simulink model "gm_combinedTxRx_ExternalMode"  (R2017b)
settings: Solver=FixedStepDiscrete  StartTime=0.0  StopTime=10.0  RelTol=1e-3
InitFcn:
  | modelSettings
undefined symbols (not defined in the file or in its folder): coeff, filt, j, RadioSampleRate, VibertiTracebackLength, xPreambleSeq
libraries: simulink x20, dsphdlfiltering x20, hdlsllib x10, hdlmdlgenlib x6, dspsigops x5, commseqgen3 x4, commdigbbndpm3 x3, commcrc2 x2, commcnvcod2 x2, commsource2 x1, dspstat3 x1, dspmlti4 x1
(part 2 of 5)

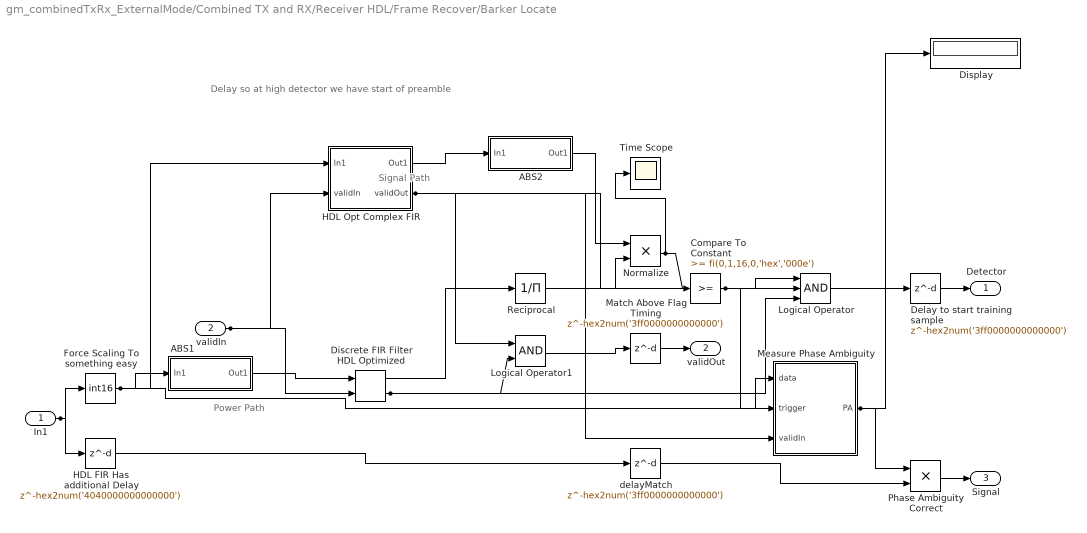
== system gm_combinedTxRx_ExternalMode/Combined TX and RX/Receiver HDL/Frame Recover/Barker Locate ==
  note: Signal Path
  note: Power Path
  note: Delay so at high detector we have start of preamble
  In1 : Inport  PortDimensions=1  SampleTime=1e-06
  validIn : Inport  Port=2  PortDimensions=1  SampleTime=1e-06
  ABS1 : Subsystem
  ABS2 : Subsystem
  Compare To Constant : simulink/Logic and Bit Operations/Compare To Constant  relop=>=  const=fi(0,1,16,0,'hex','000e')  OutDataTypeStr=boolean
  "Delay to start training sample " : Delay  DelayLength=hex2num('3ff0000000000000')  InitialCondition=0  InputProcessing=Inherited  SampleTime=1e-06
  Discrete FIR Filter HDL Optimized : dsphdlfiltering/Discrete FIR Filter HDL Optimized  Numerator=ones(1,length(xPreambleSeq)*1)/1  Sharing=off  SharingFactor=2  SimulateUsing=Code generation  roundingMode=Floor  overflowMode=off  CoefficientsDataTypeStr=Inherit: Same word length as input  CoefficientsMin=[]  CoefficientsMax=[]  OutputDataTypeStr=fixdt(1,17,0)  OutputMin=[]  OutputMax=[]  ValidInPort=on  ReadyPort=off
      settings: SourceProductName=DSP System Toolbox  SourceProductBaseCode=DS
  Display : Display
  Force Scaling To something easy : DataTypeConversion  OutDataTypeStr=int16  SampleTime=1e-06  SaturateOnIntegerOverflow=on
  HDL FIR Has additional Delay : Delay  DelayLength=hex2num('4040000000000000')  InitialCondition=0  InputProcessing=Inherited  SampleTime=1e-06
  HDL Opt Complex FIR : Subsystem  mask{Taps=reshape([complex(-0.7071067811865477, -0.7071067811865475) complex(-0.7071067811865477, -0.7071067811865475) complex(-0.7071067811865477, -0.7071067811865475) complex(0.7071067811865476, 0.7071067811865476) complex(0.7071067811865476, 0.7071067811865476) complex(0.7071067811865476, 0.7071067811865476) complex(-0.7071067811865477, -0.7071067811865475) complex(0.7071067811865476, 0.7071067811865476) complex(-0.7071067811865477, -0.7071067811865475) complex(-0.7071067811865477, -0.7071067811865475) complex(0.7071067811865476, 0.7071067811865476) complex(-0.7071067811865477, -0.7071067811865475) complex(-0.7071067811865477, -0.7071067811865475) complex(-0.7071067811865477, -0.7071067811865475) complex(0.7071067811865476, 0.7071067811865476) complex(0.7071067811865476, 0.7071067811865476) complex(0.7071067811865476, 0.7071067811865476) complex(-0.7071067811865477, -0.7071067811865475) complex(0.7071067811865476, 0.7071067811865476) complex(-0.7071067811865477, -0.7071067811865475) complex(-0.7071067811865477, -0.7071067811865475) complex(0.7071067811865476, 0.7071067811865476) complex(-0.7071067811865477, -0.7071067811865475) complex(-0.7071067811865477, -0.7071067811865475) complex(-0.7071067811865477, -0.7071067811865475) complex(0.7071067811865476, 0.7071067811865476) complex(0.7071067811865476, 0.7071067811865476) complex(0.7071067811865476, 0.7071067811865476)].', [1  28])}
  Logical Operator : Logic  Inputs=3  AllPortsSameDT=off  OutDataTypeStr=boolean  SampleTime=1e-06
  Logical Operator1 : Logic  AllPortsSameDT=off  OutDataTypeStr=boolean  SampleTime=1e-06
  Match Above Flag Timing : Delay  DelayLength=hex2num('3ff0000000000000')  InitialCondition=0  InputProcessing=Inherited  SampleTime=1e-06
  Measure Phase Ambiguity : Subsystem
  Normalize : Product  Inputs=**  OutDataTypeStr=int16  RndMeth=Simplest  SampleTime=1e-06  SaturateOnIntegerOverflow=on
  Phase Ambiguity Correct : Product  Inputs=**  OutDataTypeStr=fixdt(1, 16, 14)  SampleTime=1e-06
  Reciprocal : Product  Inputs=/  OutDataTypeStr=fixdt(1, 17, 15)  SampleTime=1e-06  SaturateOnIntegerOverflow=on  RndMeth=Zero
  Time Scope : Scope
  delayMatch : Delay  DelayLength=hex2num('3ff0000000000000')  InitialCondition=0  InputProcessing=Inherited  SampleTime=1e-06
  Detector : Outport
  validOut : Outport  Port=2
  Signal : Outport  Port=3
  wires:
  ABS1/1(Out1) -> Discrete FIR Filter HDL Optimized/1
  ABS2/1(Out1) -> Normalize/1
  Compare To Constant/1 -> Logical Operator/1, Measure Phase Ambiguity/2(trigger)
  "Delay to start training sample "/1 -> Detector/1
  Discrete FIR Filter HDL Optimized/1 -> Reciprocal/1
  Discrete FIR Filter HDL Optimized/2 -> Logical Operator1/2, Logical Operator/3
  Force Scaling To something easy/1 -> ABS1/1(In1), HDL Opt Complex FIR/1(In1), Measure Phase Ambiguity/1(data)
  delayMatch/1 -> Phase Ambiguity Correct/2
  HDL Opt Complex FIR/1(Out1) -> ABS2/1(In1)
  HDL Opt Complex FIR/2(validOut) -> Logical Operator1/1, Logical Operator/2, Measure Phase Ambiguity/3(validIn)
  Logical Operator/1 -> "Delay to start training sample "/1
  Logical Operator1/1 -> Match Above Flag Timing/1
  Match Above Flag Timing/1 -> validOut/1
  Measure Phase Ambiguity/1(PA) -> Phase Ambiguity Correct/1, Display/1
  Normalize/1 -> Compare To Constant/1, Time Scope/1
  Phase Ambiguity Correct/1 -> Signal/1
  Reciprocal/1 -> Normalize/2
  In1/1 -> Force Scaling To something easy/1, HDL FIR Has additional Delay/1
  validIn/1 -> HDL Opt Complex FIR/2(validIn), Discrete FIR Filter HDL Optimized/2
  HDL FIR Has additional Delay/1 -> delayMatch/1

== system gm_combinedTxRx_ExternalMode/Combined TX and RX/Receiver HDL/Frame Recover/Enable Equalizer and Packet Decode (Latch) ==
  start : Inport  SampleTime=1e-06
  validIn : Inport  Port=2  SampleTime=1e-06
  RxTxFixedPointLibrary_c12_Enable_Equalizer_and_Packet_Decode__L : MATLAB Function  TreatAsAtomicUnit=on
  enable : Outport
  wires:
  RxTxFixedPointLibrary_c12_Enable_Equalizer_and_Packet_Decode__L/1(enable) -> enable/1
  start/1 -> RxTxFixedPointLibrary_c12_Enable_Equalizer_and_Packet_Decode__L/1(start)
  validIn/1 -> RxTxFixedPointLibrary_c12_Enable_Equalizer_and_Packet_Decode__L/2(validIn)

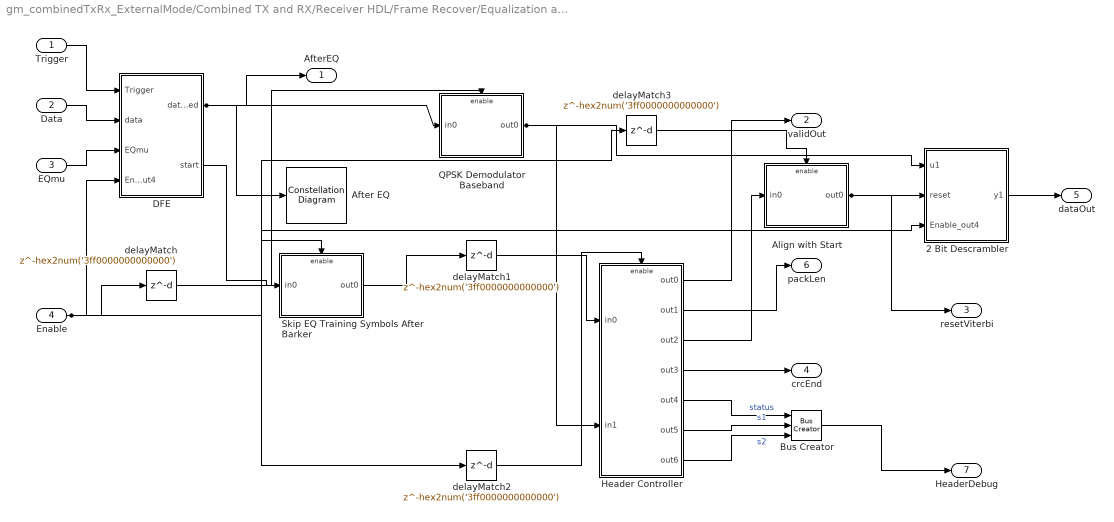
== system gm_combinedTxRx_ExternalMode/Combined TX and RX/Receiver HDL/Frame Recover/Equalization and Demodulation ==
  Trigger : Inport  SampleTime=1e-06
  Data : Inport  Port=2  SampleTime=1e-06
  EQmu : Inport  Port=3  SampleTime=1e-06
  Enable : Inport  Port=4  OutDataTypeStr=boolean  SampleTime=1e-06
  2 Bit Descrambler : Subsystem  mask{polynom=reshape([hex2num('3ff0000000000000') hex2num('3ff0000000000000') hex2num('0000000000000000') hex2num('3ff0000000000000') hex2num('0000000000000000') hex2num('3ff0000000000000') hex2num('0000000000000000') hex2num('3ff0000000000000')].', [1  8]), initstate=reshape([hex2num('0000000000000000') hex2num('3ff0000000000000') hex2num('0000000000000000') hex2num('0000000000000000') hex2num('0000000000000000') hex2num('3ff0000000000000') hex2num('0000000000000000')].', [1  7])}
      mask prompts: polynom "Polynomial"; initstate "Inital State"
      mask Display: fprintf('HDL Descrambler')
  After EQ : ConstellationDiagram
  Align with Start : Subsystem
      settings: MinAlgLoopOccurrences=on
  Bus Creator : BusCreator  Inputs=3
  DFE : Subsystem
  Header Controller : Subsystem
      settings: MinAlgLoopOccurrences=on
  QPSK Demodulator Baseband : Subsystem
      settings: MinAlgLoopOccurrences=on
  Skip EQ Training Symbols After Barker : Subsystem
      settings: MinAlgLoopOccurrences=on
  delayMatch{,1..3} (4 alike) : Delay  DelayLength=hex2num('3ff0000000000000')  InitialCondition=0  InputProcessing=Inherited
  AfterEQ : Outport  InitialOutput=0
  validOut : Outport  Port=2  InitialOutput=0
  resetViterbi : Outport  Port=3  InitialOutput=0
  crcEnd : Outport  Port=4  InitialOutput=0
  dataOut : Outport  Port=5  InitialOutput=0
  packLen : Outport  Port=6  InitialOutput=0
  HeaderDebug : Outport  Port=7  InitialOutput=0
  wires:
  delayMatch/1 -> QPSK Demodulator Baseband/Enable
  2 Bit Descrambler/1(y1) -> dataOut/1
  Align with Start/1(out0) -> 2 Bit Descrambler/2(reset), resetViterbi/1
  Bus Creator/1 -> HeaderDebug/1
  DFE/1(dataEQed) -> QPSK Demodulator Baseband/1(in0), After EQ/1, AfterEQ/1
  DFE/2(start) -> Skip EQ Training Symbols After Barker/1(in0)
  Header Controller/1(out0) -> validOut/1
  Header Controller/2(out1) -> packLen/1
  Header Controller/3(out2) -> Align with Start/1(in0)
  Header Controller/4(out3) -> crcEnd/1
  Header Controller/5(out4) -> Bus Creator/1  "status"
  Header Controller/6(out5) -> Bus Creator/2  "s1"
  Header Controller/7(out6) -> Bus Creator/3  "s2"
  QPSK Demodulator Baseband/1(out0) -> Header Controller/2(in1), 2 Bit Descrambler/1(u1)
  delayMatch1/1 -> Header Controller/1(in0)
  Trigger/1 -> DFE/1(Trigger)
  Data/1 -> DFE/2(data)
  EQmu/1 -> DFE/3(EQmu)
  Enable/1 -> delayMatch3/1, delayMatch2/1, delayMatch/1, Skip EQ Training Symbols After Barker/Enable, DFE/4(Enable_out4), 2 Bit Descrambler/3(Enable_out4)
  delayMatch2/1 -> Header Controller/Enable
  Skip EQ Training Symbols After Barker/1(out0) -> delayMatch1/1
  delayMatch3/1 -> Align with Start/Enable

== system gm_combinedTxRx_ExternalMode/Combined TX and RX/Receiver HDL/Frame Recover/Frequency Recovery ==
  note: Pull in range (Hz) = 2*pi*sqrt(2)*DampingFactor*NormLoopBandwidth*SampleRate
  note: Frequency Lock Delay = SampleRate*4*NormalizedPullInRange^2)/ (SampleRate*NormLoopBandwidth)^3;
  note: Max Phase Lock Delay= 1.3/(NormLoopBandwidth*SampleRate)
  dataIn : Inport  SampleTime=1e-06
  validIn : Inport  Port=2  SampleTime=1e-06
  LoopBW : Inport  Port=3  SampleTime=1e-06
  Enable : Inport  Port=4  OutDataTypeStr=boolean  SampleTime=1e-06
  Delay : Subsystem
      settings: MinAlgLoopOccurrences=on
  Lock Detector : Subsystem  mask{Threshold=hex2num('3f9eb851eb851eb8'), WindowLength=hex2num('4059000000000000')}
      mask prompts: WindowLength "Window Length"
  Loop Filter Configurable : Subsystem
      mask Display: disp('Loop Filter')
  PED : Subsystem
  Phase Shift FP : Subsystem
  StateControl : StateControl  StateControl=Synchronous
  dataOut : Outport  InitialOutput=0
  validOut : Outport  Port=2  InitialOutput=0
  lock : Outport  Port=3  InitialOutput=0
  wires:
  Delay/1(out0) -> dataOut/1, PED/1(In)
  Lock Detector/1(lock) -> lock/1
  PED/1(e) -> Lock Detector/1(ped), Loop Filter Configurable/1(e)
  dataIn/1 -> Phase Shift FP/1(In1)
  validIn/1 -> validOut/1
  LoopBW/1 -> Loop Filter Configurable/2(LoopBW)
  Enable/1 -> Lock Detector/2(Enable_out4), Delay/Enable, Loop Filter Configurable/3(Enable_out4)
  Loop Filter Configurable/1(v) -> Phase Shift FP/2(Phi)
  Phase Shift FP/1(Out1) -> Delay/1(in0)

== system gm_combinedTxRx_ExternalMode/Combined TX and RX/Receiver HDL/Frame Recover/Gardner Timing Recovery ==
  In1 : Inport  SampleTime=1e-06
  Enable : Inport  Port=2  OutDataTypeStr=boolean  SampleTime=1e-06
  Delay : Subsystem
      settings: MinAlgLoopOccurrences=on
  Delay1 : Subsystem
      settings: MinAlgLoopOccurrences=on
  Delay2 : Subsystem
      settings: MinAlgLoopOccurrences=on
  Gardner TED Blocks : Subsystem
  InterpControl_Blocks1 : Subsystem
  Interpolator : Subsystem
  LoopFilter1 : Subsystem  mask{zeta=hex2num('3ff6a09e667f3bcd'), BnTs=hex2num('3f847ae147ae147b'), Kp=hex2num('400599999999999a')}
      mask prompts: zeta "DampingFactor"; BnTs "NormalizedLoopBandwidth"; Kp "DetectionGain"
  StateControl : StateControl  StateControl=Synchronous
  TED Lock Detector : Subsystem  mask{Threshold=hex2num('3f847ae147ae147b'), WindowLength=hex2num('4059000000000000')}
      mask prompts: WindowLength "Window Length"
  Out1 : Outport  InitialOutput=0
  strobe : Outport  Port=2  InitialOutput=0
  lock : Outport  Port=3  InitialOutput=0
  wires:
  Delay1/1(out0) -> strobe/1, Gardner TED Blocks/2(strobe)
  Delay2/1(out0) -> Interpolator/1(In1)
  Gardner TED Blocks/1(e) -> TED Lock Detector/1(ted), LoopFilter1/1(e)
  Interpolator/1(Out1) -> Out1/1, Gardner TED Blocks/1(data)
  TED Lock Detector/1(lock) -> lock/1
  In1/1 -> Delay2/1(in0)
  Enable/1 -> Delay2/Enable, TED Lock Detector/2(Enable_out2), Delay1/Enable, Delay/Enable, LoopFilter1/2(Enable_out2), Interpolator/3(Enable_out2), InterpControl_Blocks1/2(Enable_out2), Gardner TED Blocks/3(Enable_out2)
  Delay/1(out0) -> Interpolator/2(mu)
  LoopFilter1/1(v) -> InterpControl_Blocks1/1(e)
  InterpControl_Blocks1/1(strobe) -> Delay1/1(in0)
  InterpControl_Blocks1/2(mu) -> Delay/1(in0)

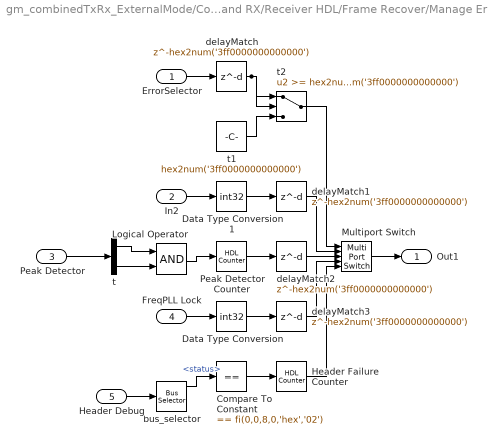
== system gm_combinedTxRx_ExternalMode/Combined TX and RX/Receiver HDL/Frame Recover/Manage Error Signals ==
  ErrorSelector : Inport  SampleTime=1e-06
  In2 : Inport  Port=2  SampleTime=1e-06
  Peak Detector : Inport  Port=3  PortDimensions=2  SampleTime=1e-06
  FreqPLL Lock : Inport  Port=4  SampleTime=1e-06
  Header Debug : Inport  Port=5  SampleTime=1e-06
  Compare To Constant : simulink/Logic and Bit Operations/Compare To Constant  relop===  const=fi(0,0,8,0,'hex','02')  OutDataTypeStr=boolean
  Data Type Conversion : DataTypeConversion  OutDataTypeStr=int32  SampleTime=1e-06
  Data Type Conversion1 : DataTypeConversion  OutDataTypeStr=int32  SampleTime=1e-06
  Header Failure Counter : hdlsllib/Sources/HDL Counter  CountType=Count limited  CountInit=hex2num('0000000000000000')  CountStep=hex2num('3ff0000000000000')  CountMax=hex2num('41efffffffe00000')  CountFromType=Initial value  CountFrom=hex2num('0000000000000000')  CountResetPort=off  CountLoadPort=off  CountEnbPort=on  CountDirPort=off  CountDataType=Unsigned  CountWordLen=32  CountFracLen=0  CountSampTime=1e-06
      settings: SourceProductBaseCode=HD
  Logical Operator : Logic  AllPortsSameDT=off  OutDataTypeStr=boolean  SampleTime=1e-06
  Multiport Switch : MultiPortSwitch  Inputs=4  DiagnosticForDefault=None  OutDataTypeStr=uint32  SampleTime=1e-06
  Peak Detector Counter : hdlsllib/Sources/HDL Counter  CountType=Count limited  CountInit=hex2num('0000000000000000')  CountStep=hex2num('3ff0000000000000')  CountMax=hex2num('41efffffffe00000')  CountFromType=Initial value  CountFrom=hex2num('0000000000000000')  CountResetPort=off  CountLoadPort=off  CountEnbPort=on  CountDirPort=off  CountDataType=Unsigned  CountWordLen=32  CountFracLen=0  CountSampTime=1e-06
      settings: SourceProductBaseCode=HD
  bus_selector : BusSelector  OutputSignals=status,s1,s2
  delayMatch{,1..3} (4 alike) : Delay  DelayLength=hex2num('3ff0000000000000')  InitialCondition=0  InputProcessing=Inherited  SampleTime=1e-06
  t : Demux  Outputs=2
  t1 : Constant  Value=hex2num('3ff0000000000000')  OutDataTypeStr=int8  SampleTime=-1
  t2 : Switch  Threshold=hex2num('3ff0000000000000')  OutDataTypeStr=int8  SampleTime=1e-06
  Out1 : Outport
  wires:
  delayMatch/1 -> t2/2, t2/1
  bus_selector/1 -> Compare To Constant/1  "<status>"
  Compare To Constant/1 -> Header Failure Counter/1
  delayMatch3/1 -> Multiport Switch/4
  delayMatch1/1 -> Multiport Switch/2
  Header Failure Counter/1 -> Multiport Switch/5
  Logical Operator/1 -> Peak Detector Counter/1
  Multiport Switch/1 -> Out1/1
  delayMatch2/1 -> Multiport Switch/3
  t/1 -> Logical Operator/1
  t/2 -> Logical Operator/2
  ErrorSelector/1 -> delayMatch/1
  In2/1 -> Data Type Conversion1/1
  Peak Detector/1 -> t/1
  FreqPLL Lock/1 -> Data Type Conversion/1
  Header Debug/1 -> bus_selector/1
  Data Type Conversion1/1 -> delayMatch1/1
  Peak Detector Counter/1 -> delayMatch2/1
  Data Type Conversion/1 -> delayMatch3/1
  t1/1 -> t2/3
  t2/1 -> Multiport Switch/1

== system gm_combinedTxRx_ExternalMode/Combined TX and RX/Receiver HDL/Frame Recover/RM: Constellation Diagram After Freq Sync ==
  In1 : Inport  SampleTime=1e-06
  Enable : EnablePort
  After Frequency Recovery : ConstellationDiagram
  wires:
  In1/1 -> After Frequency Recovery/1

== system gm_combinedTxRx_ExternalMode/Combined TX and RX/Receiver HDL/Frame Recover/RM: Constellation Diagram After SRRC ==
  In1 : Inport  SampleTime=1e-06
  Enable : EnablePort
  After SRRC : ConstellationDiagram
  wires:
  In1/1 -> After SRRC/1

== system gm_combinedTxRx_ExternalMode/Combined TX and RX/Receiver HDL/Frame Recover/RM: Constellation Diagram After Timing ==
  In1 : Inport  SampleTime=1e-06
  Enable : EnablePort
  After Timing Recovery : ConstellationDiagram
  wires:
  In1/1 -> After Timing Recovery/1

== system gm_combinedTxRx_ExternalMode/Combined TX and RX/Receiver HDL/Frame Recover/RM: Spectrum Plot From Radio ==
  In1 : Inport  SampleTime=1e-06
  Enable : EnablePort
  From Radio : SpectrumAnalyzer
  wires:
  In1/1 -> From Radio/1

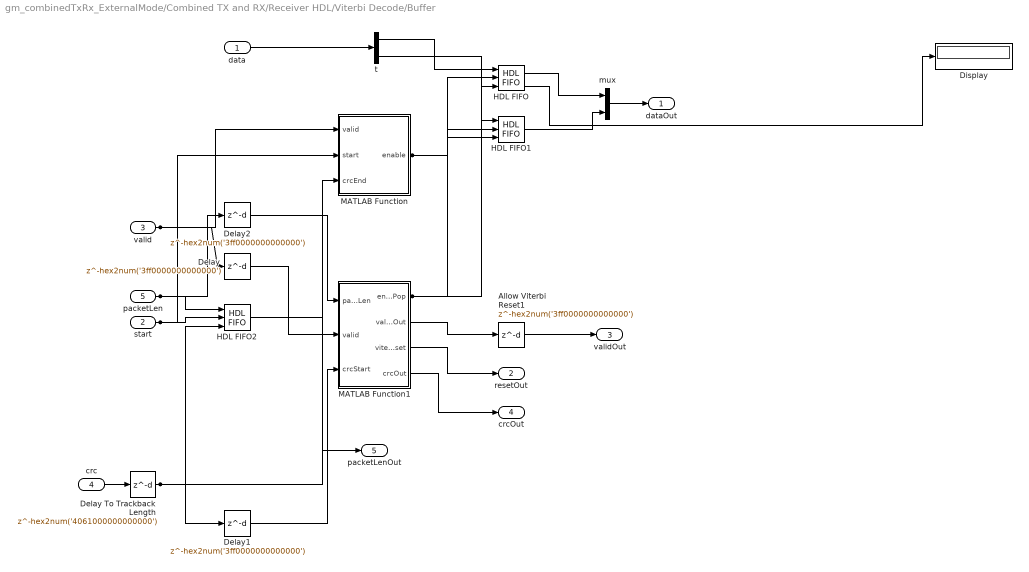
== system gm_combinedTxRx_ExternalMode/Combined TX and RX/Receiver HDL/Viterbi Decode/Buffer ==
  data : Inport  PortDimensions=2  SampleTime=1e-06
  start : Inport  Port=2  SampleTime=1e-06
  valid : Inport  Port=3  SampleTime=1e-06
  crc : Inport  Port=4  SampleTime=1e-06
  packetLen : Inport  Port=5  SampleTime=1e-06
  Allow Viterbi Reset1 : Delay  DelayLength=hex2num('3ff0000000000000')  InitialCondition=0  InputProcessing=Inherited  SampleTime=1e-06
  Delay : Delay  DelayLength=hex2num('3ff0000000000000')  InitialCondition=0  InputProcessing=Inherited  SampleTime=1e-06
  Delay To Trackback Length : Delay  DelayLength=hex2num('4061000000000000')  InitialCondition=0  InputProcessing=Inherited  SampleTime=1e-06
  Delay1 : Delay  DelayLength=hex2num('3ff0000000000000')  InitialCondition=0  InputProcessing=Inherited  SampleTime=1e-06
  Delay2 : Delay  DelayLength=hex2num('3ff0000000000000')  InitialCondition=0  InputProcessing=Inherited  SampleTime=1e-06
  Display : Display
  HDL FIFO : hdlsllib/HDL RAMs/HDL FIFO  fifo_size=2^16  ratio=1  push_msg=Warning  pop_msg=Warning  show_empty=off  show_full=off  show_num=on
      settings: SourceProductName=HDL Coder  SourceProductBaseCode=HD
  HDL FIFO1 : hdlsllib/HDL RAMs/HDL FIFO  fifo_size=2^16  ratio=1  push_msg=Warning  pop_msg=Warning  show_empty=off  show_full=off  show_num=off
      settings: SourceProductName=HDL Coder  SourceProductBaseCode=HD
  HDL FIFO2 : hdlsllib/HDL RAMs/HDL FIFO  fifo_size=2^3  ratio=1  push_msg=Warning  pop_msg=Warning  show_empty=off  show_full=off  show_num=off
      settings: SourceProductName=HDL Coder  SourceProductBaseCode=HD
  MATLAB Function : Subsystem
  MATLAB Function1 : Subsystem
  mux : Mux  Inputs=2
  t : Demux  Outputs=2
  dataOut : Outport
  resetOut : Outport  Port=2
  validOut : Outport  Port=3
  crcOut : Outport  Port=4  OutDataTypeStr=boolean
  packetLenOut : Outport  Port=5
  wires:
  Allow Viterbi Reset1/1 -> validOut/1
  Delay/1 -> MATLAB Function1/2(valid)
  Delay To Trackback Length/1 -> Delay1/1, MATLAB Function/3(crcEnd), HDL FIFO2/3
  Delay1/1 -> MATLAB Function1/3(crcStart)
  Delay2/1 -> MATLAB Function1/1(packetLen)
  HDL FIFO/1 -> mux/1
  HDL FIFO/2 -> Display/1
  HDL FIFO1/1 -> mux/2
  HDL FIFO2/1 -> packetLenOut/1
  MATLAB Function/1(enable) -> HDL FIFO/2, HDL FIFO1/2
  MATLAB Function1/1(enablePop) -> HDL FIFO/3, HDL FIFO1/3
  MATLAB Function1/2(validOut) -> Allow Viterbi Reset1/1
  MATLAB Function1/3(viterbiReset) -> resetOut/1
  MATLAB Function1/4(crcOut) -> crcOut/1
  mux/1 -> dataOut/1
  t/1 -> HDL FIFO/1
  t/2 -> HDL FIFO1/1
  data/1 -> t/1
  start/1 -> MATLAB Function/2(start), HDL FIFO2/2
  valid/1 -> Delay/1, MATLAB Function/1(valid)
  crc/1 -> Delay To Trackback Length/1
  packetLen/1 -> Delay2/1, HDL FIFO2/1

== system gm_combinedTxRx_ExternalMode/Combined TX and RX/Receiver HDL/Viterbi Decode/Viterbi Decoder ==
  In1 : Inport
  In2 : Inport  Port=2
  Viterbi Decoder : commcnvcod2/Viterbi Decoder  trellis=poly2trellis(7, [171 133])  isPunctured=off  punctureVector=[1; 1; 0; 1; 0; 1]  erasures=off  dectype=Hard decision  nsdecb=4  runSigValErrCheck=off  tbdepth=VibertiTracebackLength  opmode=Continuous  reset=on  delayedResetAction=on  smWordLength=16  outDataType=boolean
      settings: SourceProductName=Communications System Toolbox  SourceProductBaseCode=CM
  Viterbi Decoder_GenDelay1 : Delay  DelayLength=20  InputProcessing=Inherited
  Out1 : Outport
  wires:
  In1/1 -> Viterbi Decoder/1
  In2/1 -> Viterbi Decoder/2
  Viterbi Decoder/1 -> Viterbi Decoder_GenDelay1/1
  Viterbi Decoder_GenDelay1/1 -> Out1/1

== system gm_combinedTxRx_ExternalMode/Combined TX and RX/Transmitter HDL/DMA Interface/DMA Control ==
  byteIn : Inport  SampleTime=4e-06
  validIn : Inport  Port=2  SampleTime=4e-06
  EOF : Inport  Port=3  SampleTime=4e-06
  RxTxFixedPointLibrary_c18_DMA_Control : MATLAB Function  TreatAsAtomicUnit=on
  bitOut : Outport
  validOut : Outport  Port=2
  startOut : Outport  Port=3
  payloadLength : Outport  Port=4
  readyForInput : Outport  Port=5
  wires:
  byteIn/1 -> RxTxFixedPointLibrary_c18_DMA_Control/1(byteIn)
  validIn/1 -> RxTxFixedPointLibrary_c18_DMA_Control/2(validIn)
  EOF/1 -> RxTxFixedPointLibrary_c18_DMA_Control/3(EOF)
  RxTxFixedPointLibrary_c18_DMA_Control/1(bitOut) -> bitOut/1
  RxTxFixedPointLibrary_c18_DMA_Control/2(validOut) -> validOut/1
  RxTxFixedPointLibrary_c18_DMA_Control/3(startOut) -> startOut/1
  RxTxFixedPointLibrary_c18_DMA_Control/4(payloadLength) -> payloadLength/1
  RxTxFixedPointLibrary_c18_DMA_Control/5(readyForInput) -> readyForInput/1

== system gm_combinedTxRx_ExternalMode/Combined TX and RX/Transmitter HDL/Packet Generation/Payload ==
  data : Inport  SampleTime=4e-06
  start : Inport  Port=2  SampleTime=4e-06
  done : Inport  Port=3  SampleTime=4e-06
  mode : Inport  Port=4  SampleTime=4e-06
  Allow Reset : Delay  DelayLength=1
  Allow Reset of Encoder : Delay  DelayLength=1
  Compensate For Data : Delay  DelayLength=1
  Compensate For Data1 : Delay  DelayLength=1
  Compensate For Data2 : Delay  DelayLength=1
  Convolutional Encoder : commcnvcod2/Convolutional Encoder  trellis=poly2trellis(7, [171 133])  opMode=Reset on nonzero input via port  DelayedResetAction=on  hasIniStPort=off  hasFinStPort=off  usePuncVector=off  punctureVector=[1; 1; 0; 1; 0; 1]  reset=Unused parameter value
      settings: SourceProductName=Communications System Toolbox  SourceProductBaseCode=CM
  General CRC Generator HDL Optimized : commcrc2/General CRC Generator HDL Optimized  Polynomial=[1 0 0 0 0 0 1 0 0 1 1 0 0 0 0 0 1 0 0 0 1 1 1 0 1 1 0 1 1 0 1 1 1]  InitialState=0  DirectMethod=off  ReflectInput=off  ReflectCRCChecksum=off  FinalXORValue=0  SimulateUsing=Code generation
      settings: SourceProductName=Communications System Toolbox  SourceProductBaseCode=CM
  HDL Scrambler 2 bits : Subsystem  mask{poly=reshape([hex2num('3ff0000000000000') hex2num('3ff0000000000000') hex2num('0000000000000000') hex2num('3ff0000000000000') hex2num('0000000000000000') hex2num('3ff0000000000000') hex2num('0000000000000000') hex2num('3ff0000000000000')].', [1  8]), init_state=reshape([hex2num('0000000000000000') hex2num('3ff0000000000000') hex2num('0000000000000000') hex2num('0000000000000000') hex2num('0000000000000000') hex2num('3ff0000000000000') hex2num('0000000000000000')].', [1  7])}
      mask prompts: poly "Polynomial"; init_state "Initial State"
  MATLAB Function : Subsystem
  Need For Extra traceback : Delay  DelayLength=VibertiTracebackLength*2
  Random Data Gen1 : commseqgen3/PN Sequence Generator  poly='z^10 + z^7 + 1'  ini_sta=[0 0 1 0 0 1 0 0 1 1]  outBitMaskSource=Dialog parameter  shift=0  outVarSiz=off  maxOutSizeMode=Dialog parameter  maxOutSize=[10 1]  Ts=-1  sampPerFrame=1  reset=on  bitPackedOutputs=on  outDataType=double  numPackedBits=1  bitPackDataSigned=off  bitPackedOutDType=Smallest integer
      settings: SourceProductName=Communications System Toolbox
  Subsystem : Subsystem
  Switch : Switch  Criteria=u2 > Threshold
  Terminator : Terminator
  bits : Outport
  end : Outport  Port=2
  valid : Outport  Port=3
  wires:
  data/1 -> General CRC Generator HDL Optimized/1
  start/1 -> Subsystem/1(In1), General CRC Generator HDL Optimized/2
  done/1 -> Subsystem/2(In2), General CRC Generator HDL Optimized/3
  mode/1 -> Terminator/1
  Allow Reset/1 -> Switch/3
  Allow Reset of Encoder/1 -> HDL Scrambler 2 bits/2(reset)
  Compensate For Data/1 -> Need For Extra traceback/1, Compensate For Data2/1
  Compensate For Data1/1 -> valid/1
  Compensate For Data2/1 -> MATLAB Function/1(enable)
  Convolutional Encoder/1 -> HDL Scrambler 2 bits/1(bitsIn)
  General CRC Generator HDL Optimized/1 -> Allow Reset/1
  General CRC Generator HDL Optimized/2 -> Allow Reset of Encoder/1, Convolutional Encoder/2
  General CRC Generator HDL Optimized/3 -> Compensate For Data/1
  General CRC Generator HDL Optimized/4 -> Compensate For Data1/1
  HDL Scrambler 2 bits/1(bitsOut) -> bits/1
  MATLAB Function/1(reset) -> Random Data Gen1/1
  MATLAB Function/2(mode) -> Switch/2
  Need For Extra traceback/1 -> end/1
  Random Data Gen1/1 -> Switch/1
  Subsystem/1(Out1) -> General CRC Generator HDL Optimized/4
  Switch/1 -> Convolutional Encoder/1

== system gm_combinedTxRx_ExternalMode/Combined TX and RX/Transmitter HDL/Packet Generation/Preamble ==
  reset : Inport  SampleTime=4e-06
  Barker Even : LookupNDDirect  NumberOfTableDimensions=1  Table="reshape([0 0 0 0 0 0 0 0 0 0 0 0 0 0 0 0 0 0 0 0 0 0 0 0 0 0 0 0 0 0 0 0 0 0 0 0 0 0 0 0 0 0 0 0 0 0 0 0 0 0 0 0 0 0 0 0 0 0 0 0 0 0 0 0 0 0 0 0 0 0 0 0 0 0 0 0 0 0 0 0 0 0 0 0 0 0 0 0 0 0 0 0 0 0 0 0 0 0 0 0 0 0 0 0 0 0 0 0 0 0 0 0 0 0 0 0 0 0 0 0 0 0 0 0 0 0 0 0 0 0 0 0 0 0 0 0 0 0 0 0 0 0 0 0 0 0 0 0 0 0 0 0 0 0 0 0 0 0 0 0 0 0 0 0 0 0 0 0 0 0 0 0 0 0 0 0 0 0 0 0 0 0 0 0 0 0 0 0 0 0 0 0 0 0 0 0 0 0 0 0 0 0 0 0 0 0 0 0 0 0 0 0 0 0 0 0 0 0 0 0 0 0 0 0 0 0 0 0 0 0 0 0 0 0 0 0 0 0 0 0 0 0 0 0 0 0 0 0 0 0 0 0 0 0 0 0 0 0 0 0 0 0 0 0 0 0 0 0 0 0 0 0 0 0 0 0 0 0 0 0 0 0 0 0 0 0 0 0 0 0 0 0 0 0 0 0 0 0 0 0 0 0 0 0 0 0 0 0 0 0 0 0 0 0 0 0 0 0 0 0 0 0 0 0 0 0 0 0 0 0 0 0 0 0 0 0 0 0 0 0 0 0 0 0 0 0 0 0 0 0 0 0 0 0 0 0 0 0 0 0 0 0 0 0 0 0 0 0 0 0 0 0 0 0 0 0 0 0 0 0 0 0 0 0 0 0 0 0 0 0 0 0 0 0 0 0 0 0 0 0 0 0 0 0 0 0 0 0 0 0 0 0 0 0 0 0 0 0 0 0 0 0 0 0 0 0 0 0 0 0 0 0 0 0 0 0 0 0 0 0 0 0 0 0 0 0 0 0 0 0 0 0 0 0 0 0 0 0 0 0 0 0 0 0 0 0 0 0 0 0 0 0 0 0 0 0 0 0 0 0 0 0 0 0 0 0 0 0 0 0 0 0 0 0 0 0 0 0 0 0 0 0 0 0 0 0 0 0 0 0 0 0 0 0 0 0 0 0 0 0 0 0 0 0 0 0 0 0 0 0 0 0 0 0 0 0 0 0 0 0 0 0 0 0 0 0 0 0 0 0 0 0 0 0 0 0 0 0 0 0 0 0 0 0 0 0 0 0 0 0 0 0 0 0 0 0 0 0 0 0 0 0 0 0 0 0 0].', [1  587])"  DiagnosticForOutOfRangeInput=Error  SampleTime=1e-06  TableDataTypeStr=boolean
  Barker Odd : LookupNDDirect  NumberOfTableDimensions=1  Table="reshape([0 0 0 0 1 1 0 0 1 0 1 0 0 0 0 0 0 0 0 0 1 1 0 0 1 0 1 0 0 0 0 0 0 0 0 0 1 1 0 0 1 0 1 0 0 0 0 0 0 0 0 0 1 1 0 0 1 0 1 0 0 0 0 0 0 0 0 0 1 1 0 0 1 0 1 0 0 0 0 0 0 0 0 0 1 1 0 0 1 0 1 0 0 0 0 0 0 0 0 0 1 1 0 0 1 0 1 0 0 0 0 0 0 0 0 0 1 1 0 0 1 0 1 0 0 0 0 0 0 0 0 0 1 1 0 0 1 0 1 0 0 0 0 0 0 0 0 0 1 1 0 0 1 0 1 0 0 0 0 0 0 0 1 1 1 0 1 1 0 1 0 0 0 1 1 1 0 1 1 0 1 0 0 0 1 1 1 0 0 0 0 0 0 0 0 0 0 0 0 0 0 0 0 0 0 0 0 0 0 0 0 0 0 0 0 0 0 0 0 0 0 0 0 0 0 0 0 0 0 0 0 0 0 0 0 0 0 0 0 0 0 0 0 0 0 0 0 0 0 0 0 0 0 0 0 0 0 0 0 0 0 0 0 0 0 0 0 0 0 0 0 0 0 0 0 0 0 0 0 0 0 0 0 0 0 0 0 0 0 0 0 0 0 0 0 0 0 0 0 0 0 0 0 0 0 0 0 0 0 0 0 0 0 0 0 0 0 0 0 0 0 0 0 0 0 0 0 0 0 0 0 0 0 0 0 0 0 0 0 0 0 0 0 0 0 0 0 0 0 0 0 0 0 0 0 0 0 0 0 0 0 0 0 0 0 0 0 0 0 0 0 0 0 0 0 0 0 0 0 0 0 0 0 0 0 0 0 0 0 0 0 0 0 0 0 0 0 0 0 0 0 0 0 0 0 0 0 0 0 0 0 0 0 0 0 0 0 0 0 0 0 0 0 0 0 0 0 0 0 0 0 0 0 0 0 0 0 0 0 0 0 0 0 0 0 0 0 0 0 0 0 0 0 0 0 0 0 0 0 0 0 0 0 0 0 0 0 0 0 0 0 0 0 0 0 0 0 0 0 0 0 0 0 0 0 0 0 0 0 0 0 0 0 0 0 0 0 0 0 0 0 0 0 0 0 0 0 0 0 0 0 0 0 0 0 0 0 0 0 0 0 0 0 0 0 0 0 0 0 0 0 0 0 0 0 0 0 0 0 0 0 0 0 0 0 0 0 0 0 0 0 0 0 0 0 0 0 0 0 0 0 0 0 0 0 0 0 0 0 0 0 0 0 0 0 0 0 0 0 0 0 0 0 0 0 0 0].', [1  587])"  DiagnosticForOutOfRangeInput=Error  SampleTime=1e-06  TableDataTypeStr=boolean
  Delay : Delay  DelayLength=hex2num('3ff0000000000000')  InitialCondition=0  InputProcessing=Inherited  SampleTime=4e-06
  Delay1 : RateTransition  OutPortSampleTimeOpt=Multiple of input port sample time  OutPortSampleTimeMultiple=4
  Enable at end of barker : simulink/Logic and Bit Operations/Compare To Constant  relop=<  const=fi(0,0,16,0,'hex','00bb')  OutDataTypeStr=boolean
  HDL Counter : hdlsllib/Sources/HDL Counter  CountType=Count limited  CountInit=hex2num('0000000000000000')  CountStep=hex2num('3ff0000000000000')  CountMax=586  CountFromType=Initial value  CountFrom=hex2num('0000000000000000')  CountResetPort=on  CountLoadPort=off  CountEnbPort=off  CountDirPort=off  CountDataType=Unsigned  CountWordLen=16  CountFracLen=0  CountSampTime=4e-06
      settings: SourceProductBaseCode=HD
  PN Sequence For EQ : commseqgen3/PN Sequence Generator  poly='z^5 + z^3 + z^1 + 1'  ini_sta=[1 1 1 0 0]  outBitMaskSource=Dialog parameter  shift=0  outVarSiz=off  maxOutSizeMode=Dialog parameter  maxOutSize=[10 1]  Ts=-1  sampPerFrame=1  reset=on  bitPackedOutputs=on  outDataType=double  numPackedBits=2  bitPackDataSigned=off  bitPackedOutDType=Smallest integer
      settings: SourceProductName=Communications System Toolbox
  PipelineRegister : Delay  DelayLength=hex2num('3ff0000000000000')  InitialCondition=0  InputProcessing=Inherited  SampleTime=1e-06
  PipelineRegister1 : Delay  DelayLength=hex2num('3ff0000000000000')  InitialCondition=0  InputProcessing=Inherited  SampleTime=1e-06
  Reset When Barkers Are Done : simulink/Logic and Bit Operations/Compare To Constant  relop===  const=fi(0,0,16,0,'hex','00bb')  OutDataTypeStr=boolean
  Switch1 : Switch  Threshold=hex2num('3ff0000000000000')  OutDataTypeStr=boolean  SampleTime=4e-06
  Unpack1 : Subsystem
  concatenate : Concatenate
  delayMatch : Delay  DelayLength=hex2num('3ff0000000000000')  InitialCondition=0  InputProcessing=Inherited  SampleTime=4e-06
  delayMatch1 : Delay  DelayLength=hex2num('3ff0000000000000')  InitialCondition=0  InputProcessing=Inherited  SampleTime=4e-06
  inrepeat : dspsigops/Repeat  N=hex2num('4010000000000000')  RateOptions=Allow multirate processing  ic=0  mode=Unused parameter value
      settings: SourceProductName=DSP System Toolbox
  Out1 : Outport
  wires:
  reset/1 -> HDL Counter/1
  Delay/1 -> Reset When Barkers Are Done/1, inrepeat/1, Enable at end of barker/1
  delayMatch/1 -> Switch1/2
  HDL Counter/1 -> Delay/1
  PN Sequence For EQ/1 -> Unpack1/1(In1)
  Reset When Barkers Are Done/1 -> PN Sequence For EQ/1
  Switch1/1 -> Out1/1
  delayMatch1/1 -> Switch1/3
  Delay1/1 -> Switch1/1
  concatenate/1 -> Delay1/1
  inrepeat/1 -> Barker Even/1, Barker Odd/1
  PipelineRegister/1 -> concatenate/1
  PipelineRegister1/1 -> concatenate/2
  Enable at end of barker/1 -> delayMatch/1
  Unpack1/1(Out1) -> delayMatch1/1
  Barker Odd/1 -> PipelineRegister/1
  Barker Even/1 -> PipelineRegister1/1

== system gm_combinedTxRx_ExternalMode/Combined TX and RX/Transmitter HDL/Packet Generation/Random Data ==
  In1 : Inport  SampleTime=4e-06
  Random Data Gen1 : commseqgen3/PN Sequence Generator  poly='z^10 + z^7 + 1'  ini_sta=[0 0 1 0 0 1 0 0 1 1]  outBitMaskSource=Dialog parameter  shift=0  outVarSiz=off  maxOutSizeMode=Dialog parameter  maxOutSize=[10 1]  Ts=-1  sampPerFrame=1  reset=on  bitPackedOutputs=on  outDataType=double  numPackedBits=2  bitPackDataSigned=off  bitPackedOutDType=Smallest integer
      settings: SourceProductName=Communications System Toolbox
  Unpack : Subsystem
  Out1 : Outport
  wires:
  In1/1 -> Random Data Gen1/1
  Random Data Gen1/1 -> Unpack/1(In1)
  Unpack/1(Out1) -> Out1/1

== system gm_combinedTxRx_ExternalMode/Combined TX and RX/Transmitter HDL/Packet Generation/Tx Controller ==
  payloadBit : Inport  SampleTime=4e-06
  payloadSize : Inport  Port=2  SampleTime=4e-06
  count : Inport  Port=3  SampleTime=4e-06
  start : Inport  Port=4  SampleTime=4e-06
  RxTxFixedPointLibrary_c24_Tx_Controller : MATLAB Function  TreatAsAtomicUnit=on
  modeOut : Outport
  headerData : Outport  Port=2
  data : Outport  Port=3
  dataStart : Outport  Port=4
  dataEnd : Outport  Port=5
  preambleReset : Outport  Port=6
  wires:
  payloadBit/1 -> RxTxFixedPointLibrary_c24_Tx_Controller/1(payloadBit)
  payloadSize/1 -> RxTxFixedPointLibrary_c24_Tx_Controller/2(payloadSize)
  count/1 -> RxTxFixedPointLibrary_c24_Tx_Controller/3(count)
  start/1 -> RxTxFixedPointLibrary_c24_Tx_Controller/4(start)
  RxTxFixedPointLibrary_c24_Tx_Controller/1(modeOut) -> modeOut/1
  RxTxFixedPointLibrary_c24_Tx_Controller/2(headerData) -> headerData/1
  RxTxFixedPointLibrary_c24_Tx_Controller/3(data) -> data/1
  RxTxFixedPointLibrary_c24_Tx_Controller/4(dataStart) -> dataStart/1
  RxTxFixedPointLibrary_c24_Tx_Controller/5(dataEnd) -> dataEnd/1
  RxTxFixedPointLibrary_c24_Tx_Controller/6(preambleReset) -> preambleReset/1

== system gm_combinedTxRx_ExternalMode/Combined TX and RX/Receiver HDL/CRC Check and DMA Pack/DMA Interface/Bit Packer ==
  bitIn : Inport  SampleTime=1e-06
  startIn : Inport  Port=2  SampleTime=1e-06
  endIn : Inport  Port=3  SampleTime=1e-06
  err : Inport  Port=4  SampleTime=1e-06
  validIn : Inport  Port=5  SampleTime=1e-06
  RxTxFixedPointLibrary_c11_Bit_Packer : MATLAB Function  TreatAsAtomicUnit=on
  byteOut : Outport
  validOut : Outport  Port=2
  startOut : Outport  Port=3
  wires:
  RxTxFixedPointLibrary_c11_Bit_Packer/1(byteOut) -> byteOut/1
  RxTxFixedPointLibrary_c11_Bit_Packer/2(validOut) -> validOut/1
  RxTxFixedPointLibrary_c11_Bit_Packer/3(startOut) -> startOut/1
  bitIn/1 -> RxTxFixedPointLibrary_c11_Bit_Packer/1(bitIn)
  startIn/1 -> RxTxFixedPointLibrary_c11_Bit_Packer/2(startIn)
  endIn/1 -> RxTxFixedPointLibrary_c11_Bit_Packer/3(endIn)
  err/1 -> RxTxFixedPointLibrary_c11_Bit_Packer/4(err)
  validIn/1 -> RxTxFixedPointLibrary_c11_Bit_Packer/5(validIn)

== system gm_combinedTxRx_ExternalMode/Combined TX and RX/Receiver HDL/CRC Check and DMA Pack/DMA Interface/Convert Payload Length To Bytes ==
  In1 : Inport  SampleTime=1e-06
  Constant : Constant  Value=uint16(32-1)  SampleTime=-1
  Convert To Bytes From Bits : ArithShift  BitShiftNumber=3  BitShiftDirection=Right
  Convert To Uncoded : ArithShift  BitShiftNumber=1  BitShiftDirection=Right
  Data Type Conversion : DataTypeConversion  OutDataTypeStr=uint16
  Remove CRC Length : Sum  Inputs=+-  AccumDataTypeStr=uint16
  packetLengthOut : Outport
  wires:
  Constant/1 -> Remove CRC Length/2
  Convert To Bytes From Bits/1 -> Data Type Conversion/1
  Convert To Uncoded/1 -> Remove CRC Length/1
  Data Type Conversion/1 -> packetLengthOut/1
  Remove CRC Length/1 -> Convert To Bytes From Bits/1
  In1/1 -> Convert To Uncoded/1

== system gm_combinedTxRx_ExternalMode/Combined TX and RX/Receiver HDL/Frame Recover/Barker Locate/ABS1 ==
  In1 : Inport  SampleTime=1e-06
  Add : Sum
  Complex to Real-Imag : ComplexToRealImag
  Product : Product  OutDataTypeStr=int16
  Product1 : Product  OutDataTypeStr=int16
  Out1 : Outport
  wires:
  Add/1 -> Out1/1
  Complex to Real-Imag/1 -> Product/2, Product/1
  Complex to Real-Imag/2 -> Product1/2, Product1/1
  Product/1 -> Add/1
  Product1/1 -> Add/2
  In1/1 -> Complex to Real-Imag/1

== system gm_combinedTxRx_ExternalMode/Combined TX and RX/Receiver HDL/Frame Recover/Barker Locate/ABS2 ==
  In1 : Inport  SampleTime=1e-06
  Add : Sum  SaturateOnIntegerOverflow=on
  Complex to Real-Imag : ComplexToRealImag
  Product : Product  OutDataTypeStr=int16
  Product1 : Product  OutDataTypeStr=int16
  Out1 : Outport
  wires:
  Add/1 -> Out1/1
  Complex to Real-Imag/1 -> Product/2, Product/1
  Complex to Real-Imag/2 -> Product1/2, Product1/1
  Product/1 -> Add/1
  Product1/1 -> Add/2
  In1/1 -> Complex to Real-Imag/1

== system gm_combinedTxRx_ExternalMode/Combined TX and RX/Receiver HDL/Frame Recover/Barker Locate/HDL Opt Complex FIR ==
  In1 : Inport  SampleTime=1e-06
  validIn : Inport  Port=2  SampleTime=1e-06
  Add : Sum  AccumDataTypeStr=fixdt(1,16,0)
  Discrete FIR Filter HDL Optimized : dsphdlfiltering/Discrete FIR Filter HDL Optimized  Numerator=real(Taps)  Sharing=off  SharingFactor=2  SimulateUsing=Code generation  roundingMode=Floor  overflowMode=off  CoefficientsDataTypeStr=Inherit: Same word length as input  CoefficientsMin=[]  CoefficientsMax=[]  OutputDataTypeStr=fixdt(1,15,0)  OutputMin=[]  OutputMax=[]  ValidInPort=on  ReadyPort=off
      settings: SourceProductName=DSP System Toolbox  SourceProductBaseCode=DS
  Discrete FIR Filter HDL Optimized1 : dsphdlfiltering/Discrete FIR Filter HDL Optimized  Numerator=imag(Taps)  Sharing=off  SharingFactor=2  SimulateUsing=Code generation  roundingMode=Floor  overflowMode=off  CoefficientsDataTypeStr=Inherit: Same word length as input  CoefficientsMin=[]  CoefficientsMax=[]  OutputDataTypeStr=fixdt(1,15,0)  OutputMin=[]  OutputMax=[]  ValidInPort=on  ReadyPort=off
      settings: SourceProductName=DSP System Toolbox  SourceProductBaseCode=DS
  Logical Operator : Logic  AllPortsSameDT=off  OutDataTypeStr=boolean
  Out1 : Outport
  validOut : Outport  Port=2
  wires:
  Add/1 -> Out1/1
  Discrete FIR Filter HDL Optimized/1 -> Add/1
  Discrete FIR Filter HDL Optimized/2 -> Logical Operator/1
  Discrete FIR Filter HDL Optimized1/1 -> Add/2
  Discrete FIR Filter HDL Optimized1/2 -> Logical Operator/2
  Logical Operator/1 -> validOut/1
  In1/1 -> Discrete FIR Filter HDL Optimized/1, Discrete FIR Filter HDL Optimized1/1
  validIn/1 -> Discrete FIR Filter HDL Optimized/2, Discrete FIR Filter HDL Optimized1/2

== system gm_combinedTxRx_ExternalMode/Combined TX and RX/Receiver HDL/Frame Recover/Barker Locate/Measure Phase Ambiguity ==
  data : Inport  OutDataTypeStr=int16  SampleTime=1e-06
  trigger : Inport  Port=2  SampleTime=1e-06
  validIn : Inport  Port=3  SampleTime=1e-06
  Find Max and Set Output Shift : Subsystem
  HDL Opt Complex FIR4 : Subsystem  mask{Taps=reshape([complex(-0.7071067811865477, -0.7071067811865475) complex(-0.7071067811865477, -0.7071067811865475) complex(-0.7071067811865477, -0.7071067811865475) complex(0.7071067811865476, 0.7071067811865476) complex(0.7071067811865476, 0.7071067811865476) complex(0.7071067811865476, 0.7071067811865476) complex(-0.7071067811865477, -0.7071067811865475) complex(0.7071067811865476, 0.7071067811865476) complex(-0.7071067811865477, -0.7071067811865475) complex(-0.7071067811865477, -0.7071067811865475) complex(0.7071067811865476, 0.7071067811865476) complex(-0.7071067811865477, -0.7071067811865475) complex(-0.7071067811865477, -0.7071067811865475) complex(-0.7071067811865477, -0.7071067811865475) complex(0.7071067811865476, 0.7071067811865476) complex(0.7071067811865476, 0.7071067811865476) complex(0.7071067811865476, 0.7071067811865476) complex(-0.7071067811865477, -0.7071067811865475) complex(0.7071067811865476, 0.7071067811865476) complex(-0.7071067811865477, -0.7071067811865475) complex(-0.7071067811865477, -0.7071067811865475) complex(0.7071067811865476, 0.7071067811865476) complex(-0.7071067811865477, -0.7071067811865475) complex(-0.7071067811865477, -0.7071067811865475) complex(-0.7071067811865477, -0.7071067811865475) complex(0.7071067811865476, 0.7071067811865476) complex(0.7071067811865476, 0.7071067811865476) complex(0.7071067811865476, 0.7071067811865476)].', [1  28])}
  HDL Opt Complex FIR5 : Subsystem  mask{Taps=reshape([complex(-0.7071067811865475, 0.7071067811865477) complex(-0.7071067811865475, 0.7071067811865477) complex(-0.7071067811865475, 0.7071067811865477) complex(0.7071067811865476, -0.7071067811865476) complex(0.7071067811865476, -0.7071067811865476) complex(0.7071067811865476, -0.7071067811865476) complex(-0.7071067811865475, 0.7071067811865477) complex(0.7071067811865476, -0.7071067811865476) complex(-0.7071067811865475, 0.7071067811865477) complex(-0.7071067811865475, 0.7071067811865477) complex(0.7071067811865476, -0.7071067811865476) complex(-0.7071067811865475, 0.7071067811865477) complex(-0.7071067811865475, 0.7071067811865477) complex(-0.7071067811865475, 0.7071067811865477) complex(0.7071067811865476, -0.7071067811865476) complex(0.7071067811865476, -0.7071067811865476) complex(0.7071067811865476, -0.7071067811865476) complex(-0.7071067811865475, 0.7071067811865477) complex(0.7071067811865476, -0.7071067811865476) complex(-0.7071067811865475, 0.7071067811865477) complex(-0.7071067811865475, 0.7071067811865477) complex(0.7071067811865476, -0.7071067811865476) complex(-0.7071067811865475, 0.7071067811865477) complex(-0.7071067811865475, 0.7071067811865477) complex(-0.7071067811865475, 0.7071067811865477) complex(0.7071067811865476, -0.7071067811865476) complex(0.7071067811865476, -0.7071067811865476) complex(0.7071067811865476, -0.7071067811865476)].', [1  28])}
  HDL Opt Complex FIR6 : Subsystem  mask{Taps=reshape([complex(0.7071067811865476, 0.7071067811865476) complex(0.7071067811865476, 0.7071067811865476) complex(0.7071067811865476, 0.7071067811865476) complex(-0.7071067811865475, -0.7071067811865477) complex(-0.7071067811865475, -0.7071067811865477) complex(-0.7071067811865475, -0.7071067811865477) complex(0.7071067811865476, 0.7071067811865476) complex(-0.7071067811865475, -0.7071067811865477) complex(0.7071067811865476, 0.7071067811865476) complex(0.7071067811865476, 0.7071067811865476) complex(-0.7071067811865475, -0.7071067811865477) complex(0.7071067811865476, 0.7071067811865476) complex(0.7071067811865476, 0.7071067811865476) complex(0.7071067811865476, 0.7071067811865476) complex(-0.7071067811865475, -0.7071067811865477) complex(-0.7071067811865475, -0.7071067811865477) complex(-0.7071067811865475, -0.7071067811865477) complex(0.7071067811865476, 0.7071067811865476) complex(-0.7071067811865475, -0.7071067811865477) complex(0.7071067811865476, 0.7071067811865476) complex(0.7071067811865476, 0.7071067811865476) complex(-0.7071067811865475, -0.7071067811865477) complex(0.7071067811865476, 0.7071067811865476) complex(0.7071067811865476, 0.7071067811865476) complex(0.7071067811865476, 0.7071067811865476) complex(-0.7071067811865475, -0.7071067811865477) complex(-0.7071067811865475, -0.7071067811865477) complex(-0.7071067811865475, -0.7071067811865477)].', [1  28])}
  HDL Opt Complex FIR7 : Subsystem  mask{Taps=reshape([complex(0.7071067811865476, -0.7071067811865476) complex(0.7071067811865476, -0.7071067811865476) complex(0.7071067811865476, -0.7071067811865476) complex(-0.7071067811865477, 0.7071067811865475) complex(-0.7071067811865477, 0.7071067811865475) complex(-0.7071067811865477, 0.7071067811865475) complex(0.7071067811865476, -0.7071067811865476) complex(-0.7071067811865477, 0.7071067811865475) complex(0.7071067811865476, -0.7071067811865476) complex(0.7071067811865476, -0.7071067811865476) complex(-0.7071067811865477, 0.7071067811865475) complex(0.7071067811865476, -0.7071067811865476) complex(0.7071067811865476, -0.7071067811865476) complex(0.7071067811865476, -0.7071067811865476) complex(-0.7071067811865477, 0.7071067811865475) complex(-0.7071067811865477, 0.7071067811865475) complex(-0.7071067811865477, 0.7071067811865475) complex(0.7071067811865476, -0.7071067811865476) complex(-0.7071067811865477, 0.7071067811865475) complex(0.7071067811865476, -0.7071067811865476) complex(0.7071067811865476, -0.7071067811865476) complex(-0.7071067811865477, 0.7071067811865475) complex(0.7071067811865476, -0.7071067811865476) complex(0.7071067811865476, -0.7071067811865476) complex(0.7071067811865476, -0.7071067811865476) complex(-0.7071067811865477, 0.7071067811865475) complex(-0.7071067811865477, 0.7071067811865475) complex(-0.7071067811865477, 0.7071067811865475)].', [1  28])}
  Logical Operator : Logic  Inputs=5  AllPortsSameDT=off  OutDataTypeStr=boolean
  PA : Outport  InitialOutput=0
  wires:
  Find Max and Set Output Shift/1(Out1) -> PA/1
  HDL Opt Complex FIR4/1(Out1) -> Find Max and Set Output Shift/1(In1)
  HDL Opt Complex FIR4/2(validOut) -> Logical Operator/1
  HDL Opt Complex FIR5/1(Out1) -> Find Max and Set Output Shift/2(In2)
  HDL Opt Complex FIR5/2(validOut) -> Logical Operator/2
  HDL Opt Complex FIR6/1(Out1) -> Find Max and Set Output Shift/3(In4)
  HDL Opt Complex FIR6/2(validOut) -> Logical Operator/3
  HDL Opt Complex FIR7/1(Out1) -> Find Max and Set Output Shift/4(In5)
  HDL Opt Complex FIR7/2(validOut) -> Logical Operator/4
  Logical Operator/1 -> Find Max and Set Output Shift/5(Enable)
  data/1 -> HDL Opt Complex FIR4/1(In1), HDL Opt Complex FIR5/1(In1), HDL Opt Complex FIR7/1(In1), HDL Opt Complex FIR6/1(In1)
  trigger/1 -> Logical Operator/5
  validIn/1 -> HDL Opt Complex FIR4/2(validIn), HDL Opt Complex FIR5/2(validIn), HDL Opt Complex FIR7/2(validIn), HDL Opt Complex FIR6/2(validIn)

== system gm_combinedTxRx_ExternalMode/Combined TX and RX/Receiver HDL/Frame Recover/Equalization and Demodulation/2 Bit Descrambler ==
  note: This is a special Descrambler which can process 2 bits at a time
  u1 : Inport  PortDimensions=2  SampleTime=1e-06
  reset : Inport  Port=2  SampleTime=1e-06
  Enable_out4 : Inport  Port=3  OutDataTypeStr=boolean  SampleTime=1e-06
  MATLAB Function : Subsystem
      settings: MinAlgLoopOccurrences=on
  Selector1 : Selector  SampleTime=1e-06  IndexOptions=Index vector (dialog)  Indices=[hex2num('3ff0000000000000') hex2num('4008000000000000') hex2num('4014000000000000') hex2num('401c000000000000')]  OutputSizes=hex2num('3ff0000000000000')
  Selector2 : Selector  SampleTime=1e-06  IndexOptions=Index vector (dialog)  Indices=[hex2num('3ff0000000000000') hex2num('4008000000000000') hex2num('4014000000000000') hex2num('401c000000000000')]  OutputSizes=hex2num('3ff0000000000000')
  delayMatch : Delay  DelayLength=hex2num('3ff0000000000000')  InitialCondition=0  InputProcessing=Inherited
  input_xor1 : Logic  Operator=XOR  AllPortsSameDT=off  OutDataTypeStr=boolean  SampleTime=1e-06
  input_xor2 : Logic  Operator=XOR  AllPortsSameDT=off  OutDataTypeStr=boolean  SampleTime=1e-06
  mux : Mux  Inputs=2
  state_xor1 : Logic  Operator=XOR  Inputs=1  AllPortsSameDT=off  OutDataTypeStr=boolean  SampleTime=1e-06
  state_xor2 : Logic  Operator=XOR  Inputs=1  AllPortsSameDT=off  OutDataTypeStr=boolean  SampleTime=1e-06
  t : Demux  Outputs=2
  u1_0_wire : hdlmdlgenlib/Buffer
      settings: SourceProductName=HDL Coder  SourceProductBaseCode=HD
  u1_1_wire : hdlmdlgenlib/Buffer
      settings: SourceProductName=HDL Coder  SourceProductBaseCode=HD
  y1 : Outport  InitialOutput=0
  wires:
  u1_0_wire/1 -> input_xor1/2
  u1_1_wire/1 -> input_xor2/2
  MATLAB Function/1(out0) -> Selector1/1
  MATLAB Function/2(out1) -> Selector2/1
  mux/1 -> y1/1
  Selector1/1 -> state_xor1/1
  Selector2/1 -> state_xor2/1
  input_xor1/1 -> mux/1
  input_xor2/1 -> mux/2
  state_xor1/1 -> input_xor1/1
  state_xor2/1 -> input_xor2/1
  delayMatch/1 -> MATLAB Function/Enable
  t/1 -> u1_0_wire/1
  t/2 -> u1_1_wire/1
  u1/1 -> t/1, MATLAB Function/1(in0)
  reset/1 -> MATLAB Function/2(in1)
  Enable_out4/1 -> delayMatch/1

== system gm_combinedTxRx_ExternalMode/Combined TX and RX/Receiver HDL/Frame Recover/Equalization and Demodulation/Align with Start ==
  in0 : Inport  OutDataTypeStr=boolean  SampleTime=1e-06
  Enable_out4 : EnablePort  OutDataTypeStr=boolean
  Align with Start : Delay  DelayLength=hex2num('3ff0000000000000')  InitialCondition=0  InputProcessing=Inherited
  out0 : Outport  OutDataTypeStr=boolean  InitialOutput=0
  wires:
  Align with Start/1 -> out0/1
  in0/1 -> Align with Start/1

== system gm_combinedTxRx_ExternalMode/Combined TX and RX/Receiver HDL/Frame Recover/Equalization and Demodulation/DFE ==
  note: Generate training sequence when barker is found
  note: refTap=0 to disableEQ
  Trigger : Inport  PortDimensions=1  SampleTime=1e-06
  data : Inport  Port=2  PortDimensions=1  SampleTime=1e-06
      settings: SignalType=complex
  EQmu : Inport  Port=3  SampleTime=1e-06
  Enable_out4 : Inport  Port=4  OutDataTypeStr=boolean  SampleTime=1e-06
  DFE : Subsystem  mask{numFTaps=hex2num('4014000000000000'), numBTaps=hex2num('4008000000000000'), mu=hex2num('3f847ae147ae147b'), refTap=hex2num('4000000000000000')}
      mask prompts: numFTaps "Num Forward Taps"; numBTaps "Num Backward Taps"; mu "Step Size"; refTap "Reference Tap"
  Delay data so DFE can reset : Subsystem
      settings: MinAlgLoopOccurrences=on
  Delay ref so DFE can reset : Subsystem
      settings: MinAlgLoopOccurrences=on
  PN Sequence Generator : Subsystem
      settings: MinAlgLoopOccurrences=on
  Packeted To Unpacked : Subsystem
  QPSK Modulator Baseband : Subsystem
      settings: MinAlgLoopOccurrences=on
  Terminator1 : Terminator
  delayMatch : Delay  DelayLength=hex2num('3ff0000000000000')  InitialCondition=0  InputProcessing=Inherited
  dataEQed : Outport  InitialOutput=0
  start : Outport  Port=2  InitialOutput=0
  wires:
  DFE/1(eqOut) -> dataEQed/1
  DFE/2(err) -> Terminator1/1
  DFE/3(start) -> start/1
  Delay data so DFE can reset/1(out0) -> DFE/2(dataIn)
  Delay ref so DFE can reset/1(out0) -> DFE/3(training)
  PN Sequence Generator/1(out0) -> Packeted To Unpacked/1(In1)
  Packeted To Unpacked/1(Out1) -> QPSK Modulator Baseband/1(in0)
  QPSK Modulator Baseband/1(out0) -> Delay ref so DFE can reset/1(in0)
  delayMatch/1 -> Delay data so DFE can reset/Enable
  Trigger/1 -> PN Sequence Generator/1(in0), DFE/1(reset)
  data/1 -> Delay data so DFE can reset/1(in0)
  EQmu/1 -> DFE/4(EQmu)
  Enable_out4/1 -> delayMatch/1, QPSK Modulator Baseband/Enable, PN Sequence Generator/Enable, Delay ref so DFE can reset/Enable, DFE/5(Enable_out4)
